simulink model "Yaw_try1"  (R2024b)
settings: Solver=VariableStepAuto  StartTime=0.0  StopTime=10  RelTol=1e-3
settings Model: Creator=admin  LastModifiedBy=admin

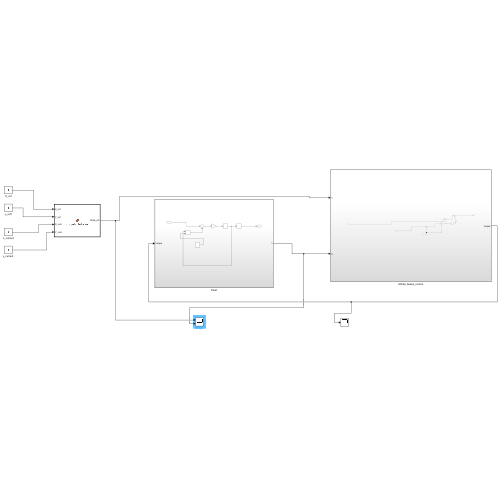
[thumbnail: Simulink's stored preview of the top-level diagram]
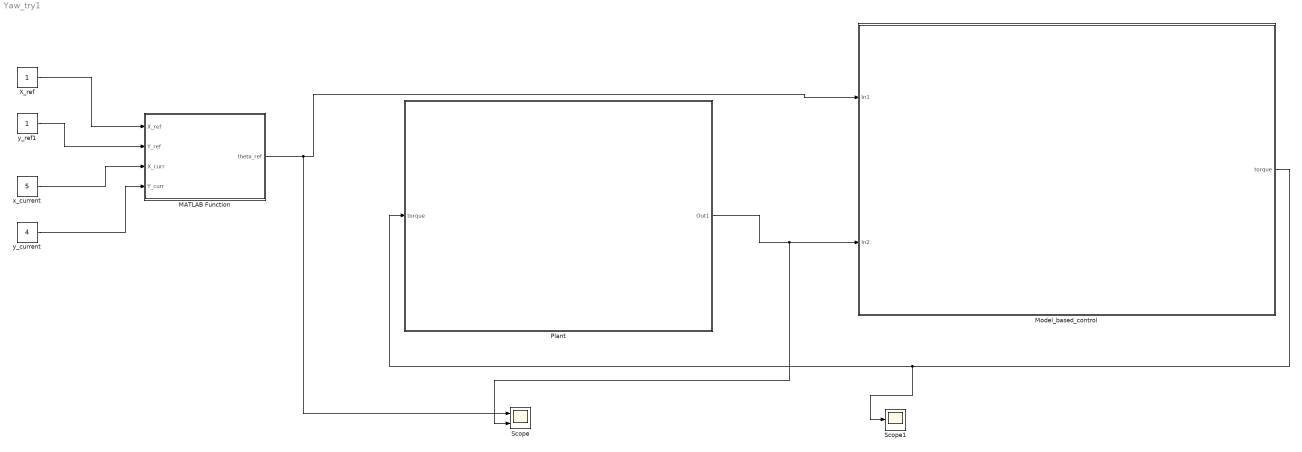
== system Yaw_try1 ==
  MATLAB Function : MATLAB Function  TreatAsAtomicUnit=on
  Model_based_control : Subsystem
  Plant : Subsystem
  Scope : Scope  NumInputPorts=2
  Scope1 : Scope
  X_ref : Constant
  x_current : Constant  Value=5
  "y_current " : Constant  Value=4
  y_ref1 : Constant
  wires:
  X_ref/1 -> MATLAB Function/1(X_ref)
  y_ref1/1 -> MATLAB Function/2(Y_ref)
  x_current/1 -> MATLAB Function/3(X_curr)
  "y_current "/1 -> MATLAB Function/4(Y_curr)
  MATLAB Function/1(theta_ref) -> Scope/1, Model_based_control/1(In1)
  Plant/1(Out1) -> Scope/2, Model_based_control/2(In2)
  Model_based_control/1(torque) -> Scope1/1, Plant/1(torque)

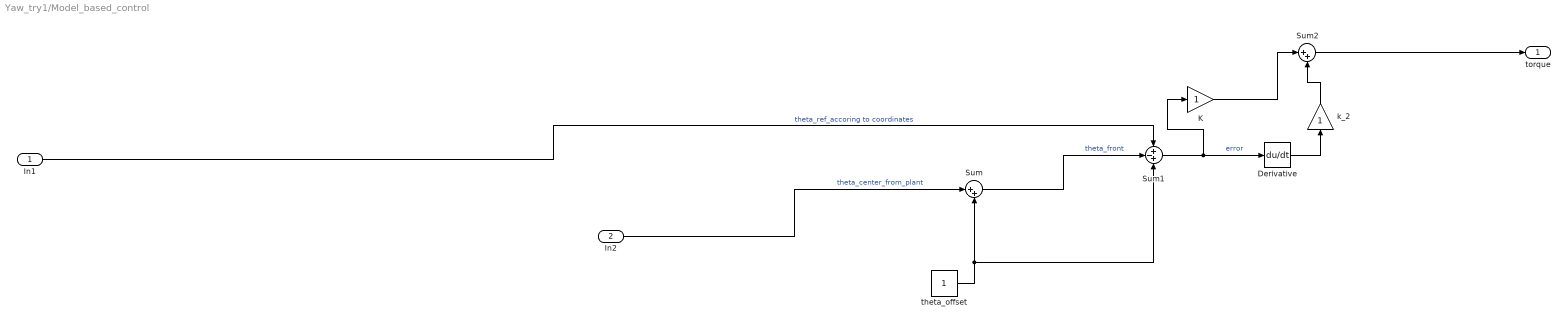
== system Yaw_try1/Model_based_control ==
  In1 : Inport
  In2 : Inport  Port=2
  Derivative : Derivative
  K : Gain
  Sum : Sum  Inputs=|++
  Sum1 : Sum  Inputs=+-+
  Sum2 : Sum  Inputs=|++
  k_2 : Gain
  theta_offset : Constant
  torque : Outport
  wires:
  Sum/1 -> Sum1/2  "theta_front"
  In2/1 -> Sum/1  "theta_center_from_plant"
  In1/1 -> Sum1/1  "theta_ref_accoring to coordinates"
  Sum1/1 -> K/1, Derivative/1  "error"
  K/1 -> Sum2/1
  Derivative/1 -> k_2/1
  k_2/1 -> Sum2/2
  Sum2/1 -> torque/1
  theta_offset/1 -> Sum1/3, Sum/2

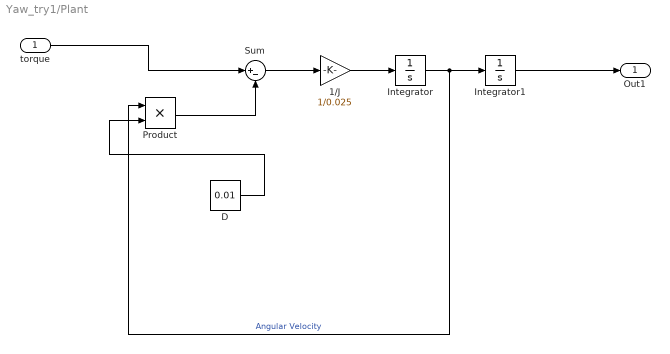
== system Yaw_try1/Plant ==
  torque : Inport
  1/J : Gain  Gain=1/0.025
  D : Constant  Value=0.01
  Integrator : Integrator
  Integrator1 : Integrator
  Product : Product
  Sum : Sum  Inputs=|+-
  Out1 : Outport
  wires:
  Product/1 -> Sum/2
  D/1 -> Product/2
  Sum/1 -> 1/J/1
  torque/1 -> Sum/1
  Integrator/1 -> Integrator1/1, Product/1  "Angular Velocity"
  1/J/1 -> Integrator/1
  Integrator1/1 -> Out1/1

== matlab function Yaw_try1/MATLAB Function ==
  data: X_ref input; theta_ref output; Y_ref input; X_curr input; Y_curr input
function theta_ref = compute_theta_ref(X_ref,Y_ref,X_curr,Y_curr)
% returns angle from current position to reference
theta_ref = atan2(Y_ref - Y_curr, X_ref - X_curr);
end
